simulink model "tp3ejercicio8"  (R2021a)
settings: Solver=VariableStepAuto  StartTime=0.0  StopTime=10.0  RelTol=1e-3
undefined symbols (not defined in the file or in its folder): gray, Rec, SDTV
libraries: visionconversions x2, visionsources x1
settings Model: Creator=ZeK005  LastModifiedBy=ZeK005

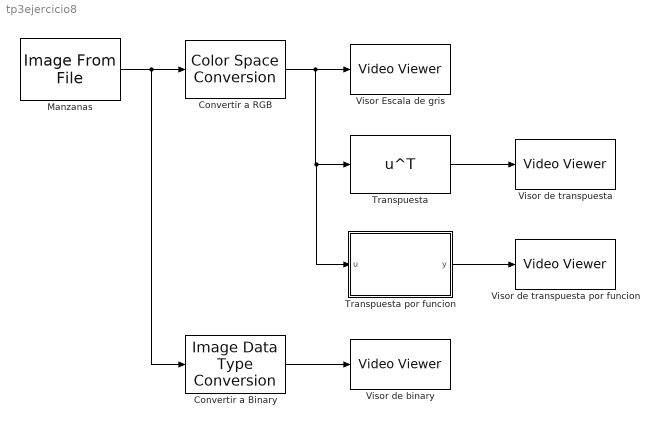
== system tp3ejercicio8 ==
  Convertir a Binary : visionconversions/Image Data Type Conversion  outDT=boolean  isSigned=on  wordLen=16  numFracBits=0
      settings: SourceProductBaseCode=VP
  Convertir a RGB : visionconversions/Color Space  Conversion  conversion=Obsolete  conversionActive=R'G'B' to intensity  wp_str=D65  rec=Rec. 601 (SDTV)  sys=1125/60/2:1  imagePorts=One multidimensional signal
  Manzanas : visionsources/Image From File  Tag=vipblks_nd  FileName=C:\Users\ZeK005\Desktop\FRT UTN\Proyectos\Matlab\2024\PDI\manzanas.jpg  Ts=inf  imagePorts=One multidimensional signal  OutPortLabels=R|G|B  ImageDataType=Inherit from input image  sdImageDataType=uint(8)  Signed=on  WordLength=16  FractionLengthMode=User-defined  FractionLength=15
  Transpuesta : Math  Operator=transpose  SaturateOnIntegerOverflow=on
  Transpuesta por funcion : MATLAB Function  TreatAsAtomicUnit=on
  Visor Escala de gris : VideoViewer  colormapValue=gray(256)  FigPos=[2 513 666 405]
  Visor de binary : VideoViewer  colormapValue=gray(256)  FigPos=[2 1029 666 405]
  Visor de transpuesta : VideoViewer  colormapValue=gray(256)  FigPos=[669 513 346 405]
  Visor de transpuesta por funcion : VideoViewer  colormapValue=gray(256)  FigPos=[671 1029 344 405]
  wires:
  Convertir a RGB/1 -> Transpuesta por funcion/1(u), Transpuesta/1, Visor Escala de gris/1
  Convertir a Binary/1 -> Visor de binary/1
  Manzanas/1 -> Convertir a RGB/1, Convertir a Binary/1
  Transpuesta/1 -> Visor de transpuesta/1
  Transpuesta por funcion/1(y) -> Visor de transpuesta por funcion/1

== matlab function tp3ejercicio8/Transpuesta por funcion ==
  data: u input; y output
function y = fcn(u)
    y = u';
end
